simulink model "simnonlin"  (R2016a)
settings: Solver=FixedStepAuto  StartTime=0.0  StopTime=10.0  FixedStep=Ts  MaxStep=0.01  RelTol=1e-3
values from neighbouring files (symbols this model uses):
  b = 0.1    [funkciadynamiky.m]    (also in param.mat; simnelinkyvadlo.m; simnelinkyvadlo_mine.m)
  g = 9.81    [funkciadynamiky.m]    (also in param.mat; simnelinkyvadlo.m; simnelinkyvadlo_mine.m)
  l = 0.2    [funkciadynamiky.m]    (also in param.mat; simnelinkyvadlo.m; simnelinkyvadlo_mine.m)
  m1 = 0.4    [funkciadynamiky.m]    (also in param.mat; simnelinkyvadlo.m; simnelinkyvadlo_mine.m)
  m2 = 0.08    [funkciadynamiky.m]    (also in param.mat; simnelinkyvadlo.m; simnelinkyvadlo_mine.m)
settings Model: Creator=UAMAI-LENOVO  LastModifiedBy=gulan
settings DataIOCC: LimitDataPoints=on  SaveFormat=Array
settings HardwareCC: ProdBitPerPointer=32  ProdLargestAtomicFloat=None  ProdIntDivRoundTo=Undefined  ProdEndianess=Unspecified  ProdWordSize=32  ProdHWDeviceType=32-bit Generic
settings ModelReferenceCC: PropagateSignalLabelsOutOfModel=off
settings ConfigComp: CovModelRefEnable=Off

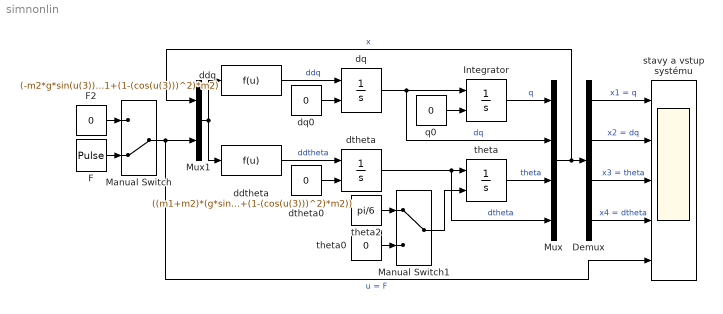
== system simnonlin ==
  " stavy a vstup systému" : Scope  NumInputPorts=5
  Demux : Demux
  F : DiscretePulseGenerator  PulseType=Time based  Amplitude=-1  Period=10  PulseWidth=0.1  PhaseDelay=0.01
  F2 : Constant  Value=0
  Integrator : Integrator  InitialConditionSource=external
  Manual Switch : ManualSwitch  CurrentSetting=0
  Manual Switch1 : ManualSwitch
  Mux : Mux
  Mux1 : Mux  Inputs=2
  ddq : Fcn  Expr=(-m2*g*sin(u(3))*cos(u(3))+m2*l*((u(4))^2)*sin(u(3))+b*m2*u(4)*cos(u(3))+u(5))/(m1+(1-(cos(u(3)))^2)*m2)
  ddtheta : Fcn  Expr=((m1+m2)*(g*sin(u(3))-b*u(4))-(m2*l*((u(4))^2)*sin(u(3))+u(5))*cos(u(3)))/(l*(m1+(1-(cos(u(3)))^2)*m2))
  dq : Integrator  InitialConditionSource=external
  dq0 : Constant  Value=0
  dtheta : Integrator  InitialConditionSource=external
  dtheta0 : Constant  Value=0
  q0 : Constant  Value=0
  theta : Integrator  InitialConditionSource=external
  theta0 : Constant  Value=0
  theta2 : Constant  Value=pi/6
  wires:
  dq/1 -> Mux/2, Integrator/1  "dq"
  dtheta/1 -> Mux/4, theta/1  "dtheta"
  Integrator/1 -> Mux/1  "q"
  theta/1 -> Mux/3  "theta"
  ddq/1 -> dq/1  "ddq"
  ddtheta/1 -> dtheta/1  "ddtheta"
  dq0/1 -> dq/2
  q0/1 -> Integrator/2
  dtheta0/1 -> dtheta/2
  Mux/1 -> Mux1/1, Demux/1  "x"
  Mux1/1 -> ddtheta/1, ddq/1
  Demux/3 -> " stavy a vstup systému"/3  "x3 = theta"
  Demux/4 -> " stavy a vstup systému"/4  "x4 = dtheta"
  Demux/1 -> " stavy a vstup systému"/1  "x1 = q"
  Demux/2 -> " stavy a vstup systému"/2  "x2 = dq"
  Manual Switch/1 -> " stavy a vstup systému"/5, Mux1/2  "u = F"
  F2/1 -> Manual Switch/1
  F/1 -> Manual Switch/2
  theta2/1 -> Manual Switch1/1
  Manual Switch1/1 -> theta/2
  theta0/1 -> Manual Switch1/2
